simulink model "generic_20231123_1032"  (R2022b)
settings: Solver=ode45  StartTime=0.0  StopTime=50  RelTol=1e-3  EnableMultiTasking=on
model workspace (MAT data in the model file):
  A = 1
  B = 1.19071237887
  kd = -9.99955278144
  ki = 0.00519416981022
  kp = 9.99999979837
undefined symbols (not defined in the file): brake_select, curvature, DiscIntNeverNeededParam, speed
libraries: CarMaker4SL x88, simulink x1, mpcadaslib x1
(part 4 of 4)

== matlab function generic_20231123_1032/CarMaker/VehicleControl/CreateBus VhclCtrl/A*algoithm/MATLAB Function1 ==
  data: start input; deviation output; target input; obstacles input; pathX output; pathY output
function [deviation, pathX, pathY] = generatePathWithObstacles(start, target, obstacles)
    % A* Path Planning
    function path = astar(start, goal, obstacles)
    % A* algorithm implementation
    
    function path = reconstructPath(parent, current)
    % Reconstruct the path from the parent array
    path_old = current;
    while any(parent(:, 1) == path_old(1) & parent(:, 2) == path_old(2))
        idx = find(parent(:, 1) == path_old(1) & parent(:, 2) == path_old(2), 1);
        path = [parent(idx, :); path_old];
    end
    path = path_old;
end
    function neighbors = generateNeighbors(current, obstacles)
    % Generate neighboring nodes (adjacent and diagonal)
    possibleMoves = [-1, 0; 1, 0; 0, -1; 0, 1; -1, -1; -1, 1; 1, -1; 1, 1];
    neighbors = bsxfun(@plus, current, possibleMoves);

    % Filter out neighbors outside the map
    inMap = neighbors(:, 1) >= 1 & neighbors(:, 1) <= 100 & neighbors(:, 2) >= 1 & neighbors(:, 2) <= 100;
    neighbors = neighbors(inMap, :);
    end
    function result = inSet(position, set)
    % Check if a position is in the set
    result = any(isequal(set(:, 1:2), position), 2);
end

    function result = inObstacles(position, obstacles)
    % Check if a position is in the obstacles
    result = any(isequal(obstacles, position), 2);
    end
    % Parameters
    mapSize = 100; % Adjust as needed
    openSet = zeros(mapSize, 3); % [x, y, f]
    closedSet = zeros(mapSize, 3); % [x, y, f]
    parent = zeros(mapSize, 2); % [parentX, parentY]

    % Functions to calculate heuristic and cost
    heuristic = @(pos, goal) sqrt((pos(1) - goal(1))^2 + (pos(2) - goal(2))^2);
    cost = @(pos, parent) sqrt((pos(1) - parent(1))^2 + (pos(2) - parent(2))^2);

    % Initialize starting point
    openSet(1, :) = [start, heuristic(start, goal)];
    closedSet = zeros(mapSize, 3);

    while any(openSet(:, 1))
        % Find the node with the lowest f in the open set
        [~, currentIdx] = min(openSet(:, 3));
        current = openSet(currentIdx, 1:2);

        % Goal reached
        if isequal(current, goal)
            path = reconstructPath(parent, current);
            return;
        end

        % Move current from openSet to closedSet
        openSet(currentIdx, :) = [0, 0, 0];
        closedSet(currentIdx, :) = [current, heuristic(current, goal)];

        % Generate neighbors
        neighbors = generateNeighbors(current, obstacles);

        for i = 1:size(neighbors, 1)
            neighbor = neighbors(i, :);

            % Skip if in closedSet or obstacle
            if ~inSet(neighbor, closedSet) && ~inObstacles(neighbor, obstacles)
                % Calculate tentative g score
                tentativeG = cost(neighbor, current) + cost(current, start);

                % Check if neighbor is not in openSet or has a better g score
                idxInOpenSet = find(isequal(openSet(:, 1:2), neighbor), 1);
                if isempty(idxInOpenSet) || tentativeG < cost(neighbor, start)
                    % Update parent and g score
                    parent(idxInOpenSet, :) = current;
                    openSet(idxInOpenSet, :) = [neighbor, tentativeG + heuristic(neighbor, goal)];
                end
            end
        end
    end

    % No path found
    path = [];
end
    path = astar(start, target, obstacles);

    % Extract X and Y coordinates from the path
    pathX1 = path(:, 1);
    pathX = pathX1(1);
    pathY1 = path(:, 2);
    pathY = pathY1(1);

    % Calculate deviation from the vehicle to the generated path
    deviation_1 = sqrt((start(1) - pathX).^2 + (start(2) - pathY).^2);
    deviation =deviation_1(1); 
end

== matlab function generic_20231123_1032/CarMaker/VehicleControl/CreateBus VhclCtrl/MATLAB Function ==
  data: x input; path_out output; y input
function path_out = fcn(x,y)
path_out = zeros(2,20);
for i=1:20
    path_out(1,i) = x+(i-10)*0.0005;
    path_out(2,i) = y+(i-10)*0.0005;
end

== matlab function generic_20231123_1032/CarMaker/VehicleControl/CreateBus VhclCtrl/Stanley_controller/Stanley/Subsystem/advanced_speed_and_brake_control ==
  data: path_curv input; throttle output; min_s_speed input; brake_cmd output; speed_act input; desired_speed input; Kd_speed input; Ki_speed input; Kp_speed input
function [throttle, brake_cmd] = advanced_speed_and_brake_control(path_curv, min_s_speed, speed_act, desired_speed,Kd_speed,Ki_speed,Kp_speed)
    persistent integrator_speed;
    persistent prev_speed_error;
    persistent integrator_brake;
    persistent prev_brake_error;

    if isempty(integrator_speed)
        integrator_speed = 0;
        prev_speed_error = 0;
        integrator_brake = 0;
        prev_brake_error = 0;
    end


   
    % Speed Control (PID)
    %disp(speed_act)
    %disp("teh speed is ")
    %disp(desired_speed)
    speed_error = desired_speed - speed_act;
    %Kp_speed = 1.900;
    %Ki_speed = 0.0300;
    %Kd_speed = 1.00;
    integrator_speed = integrator_speed + speed_error;
    derivative_speed = speed_error - prev_speed_error;
    
    throttle = Kp_speed * speed_error + Ki_speed * integrator_speed + Kd_speed * derivative_speed;

    % Braking Control (PID)
    brake_error = -speed_error;
    Kp_brake = 0.05;
    Ki_brake = 0.01;
    Kd_brake = 0.05;
    integrator_brake = integrator_brake + brake_error;
    derivative_brake = brake_error - prev_brake_error;
    brake_cmd = Kp_brake * brake_error + Ki_brake * integrator_brake + Kd_brake * derivative_brake;

    % Predictive Braking based on Path Curvature
    path_curvature = max(path_curv);
    min_safe_speed = max(min_s_speed);
    predictive_brake_factor = speed_act/100;
    if path_curvature > 0 && speed_act < min_safe_speed
        brake_cmd = brake_cmd + predictive_brake_factor * (min_safe_speed - speed_act);
    end
    % Update persistent variables
    prev_speed_error = speed_error;
    prev_brake_error = brake_error;
end

== matlab function generic_20231123_1032/CarMaker/VehicleControl/CreateBus VhclCtrl.Steering/MATLAB Function2 ==
  data: x_car input; nw_pth_gtd output; y_car input; trgt_x input; trgt_y input
function nw_pth_gtd = fcn(x_car,y_car,trgt_x,trgt_y)
nw_pth_gtd = zeros(2,1);
nw_pth_gtd(1,1) = x_car+trgt_x;
nw_pth_gtd(2,1) = y_car + trgt_y;

== matlab function generic_20231123_1032/CarMaker/VehicleControl/CreateBus VhclCtrl/Stanley_controller/MATLAB Function ==
  data: speed_rf input; throttle output; current_speed input; A input; B input
function throttle = advanced_speed_control_mpc(speed_rf, current_speed,A,B)
    % Model Predictive Controller (MPC) for speed contol
    speed_ref  = speed_rf+0.4;
    % Define MPC parameters
    Ts = 0.1;  % Sampling time
    N = 10;    % Prediction horizon
    Q = 1;     % State weight
    R = 1;     % Input weight
    S = 0.1;   % Terminal state weight (integral term)
    
    % State-space model (simplified for illustration)
    %A = 0.8;
    %B = Ts;
    
    % Define cost and constraints for fmincon
    costFunction = @(u) (current_speed - speed_ref + B * u)' * Q * (current_speed - speed_ref + B * u) + u' * R * u + S * sum(u);
    Aeq = [];
    Beq = [];
    Aineq = [];
    Bineq = [];
    lb = 0; % Lower bound on throttle
    ub = 1;  % Upper bound on throttle
    
    % Steady-state error constraint
    Aineq = [Aineq; B];
    Bineq = [Bineq; speed_ref - current_speed];
    
    % Initial guess
    u0 = 0;
    
    % Solve optimization problem
    options = optimoptions('fmincon', 'Display', 'off', 'Algorithm', 'sqp');
    u_opt = fmincon(costFunction, u0, Aineq, Bineq, Aeq, Beq, lb, ub, [], options);
    
    % Extract control input (throttle) from the optimization result
    throttle = u_opt;
end

== matlab function generic_20231123_1032/CarMaker/VehicleControl/CreateBus VhclCtrl/Subsystem3/MATLAB Function5 ==
  data: x_vehicle input; cte output; y_vehicle input; x_point input; y_point input; denominator output; x2 input; y2 input
function [cte,denominator]= calculate_cross_track_error(x_vehicle, y_vehicle, x_point, y_point,x2,y2)
    % Calculate cross-track error for a given vehicle position and single point
    function cte = calculate_perpendicular_distance(x_vehicle, y_vehicle, x_point, y_point)
    % Calculate the perpendicular distance from the vehicle to the point

    % Coordinates of the point
    x1 = x_point;
    y1 = y_point;
    %x2 = x_vehicle;
    %y2 = y_vehicle;

    % Calculate the cross-track error using the formula for the distance from a point to a line
    numerator = (x2 - x1) * (y1 - y_vehicle) - (x1 - x_vehicle) * (y2 - y1);
    denominator = sqrt((x2 - x1)^2 + (y2 - y1)^2);

    % Ensure that the denominator is not zero to avoid division by zero
    if denominator ~= 0
        cte = (numerator / denominator);
    else
        cte = 0;
    end
end
    % Calculate cross-track error as the perpendicular distance
    cte = calculate_perpendicular_distance(x_vehicle, y_vehicle, x_point, y_point);
end

== matlab function generic_20231123_1032/CarMaker/VehicleControl/CreateBus VhclCtrl/Subsystem2/MATLAB Function7 ==
  data: x_vehicle input; cte output; y_vehicle input; x_point input; y_point input; denominator output; x2 input; y2 input
function [cte,denominator]= calculate_cross_track_error(x_vehicle, y_vehicle, x_point, y_point,x2,y2)
    % Calculate cross-track error for a given vehicle position and single point
    function cte = calculate_perpendicular_distance(x_vehicle, y_vehicle, x_point, y_point)
    % Calculate the perpendicular distance from the vehicle to the point

    % Coordinates of the point
    x1 = x_point;
    y1 = y_point;
    %x2 = x_vehicle;
    %y2 = y_vehicle;

    % Calculate the cross-track error using the formula for the distance from a point to a line
    numerator = (x2 - x1) * (y1 - y_vehicle) - (x1 - x_vehicle) * (y2 - y1);
    denominator = sqrt((x2 - x1)^2 + (y2 - y1)^2);

    % Ensure that the denominator is not zero to avoid division by zero
    if denominator ~= 0
        cte = (numerator / denominator);
    else
        cte = 0;
    end
end
    % Calculate cross-track error as the perpendicular distance
    cte = calculate_perpendicular_distance(x_vehicle, y_vehicle, x_point, y_point);
end
